simulink model "quadcoptermodel"  (R2017b)
settings: Solver=FixedStepAuto  StartTime=0.0  StopTime=11  FixedStep=1/250  RelTol=1e-3
values from neighbouring files (symbols this model uses):
  a1 = (Iyy-Izz)/Ixx    (= -1)    [param_init.m]
  a2 = Jr/Ixx    (= 0.00434930232558)    [param_init.m]
  a3 = (Izz-Ixx)/Iyy    (= 1)    [param_init.m]
  a4 = Jr/Iyy    (= 0.00434930232558)    [param_init.m]
  a5 = (Ixx-Iyy)/Izz    (= 0)    [param_init.m]
  b1 = l/Ixx    (= 26.1627906977)    [param_init.m]
  b2 = l/Iyy    (= 26.1627906977)    [param_init.m]
  b3 = l/Izz    (= 13.0813953488)    [param_init.m]
  g = 9.81    [param_init.m]
  kd_Phi = 0.1969    [param_init.m]
  kd_Psi = 0.1528    [param_init.m]
  kd_Theta = 0.2022    [param_init.m]
  kd_X = .7    (= 0.7)    [param_init.m]
  kd_Y = .7    (= 0.7)    [param_init.m]
  kd_Z = 10    [param_init.m]
  kf = 3.13e-5    (= 3.13e-05)    [param_init.m]
  ki_Phi = 2.2310    (= 2.231)    [param_init.m]
  ki_Psi = 1.8013    [param_init.m]
  ki_Theta = 2.1756    [param_init.m]
  ki_X = .1    (= 0.1)    [param_init.m]
  ki_Y = .1    (= 0.1)    [param_init.m]
  ki_Z = 0    [param_init.m]
  km = 9e-7    (= 9e-07)    [param_init.m]
  kp_Phi = 2.9996    [param_init.m]
  kp_Psi = 2.479    [param_init.m]
  kp_Theta = 3.0239    [param_init.m]
  kp_X = 2    [param_init.m]
  kp_Y = 2    [param_init.m]
  kp_Z = 30    [param_init.m]
  m = 0.4794    [param_init.m]
  omega_max = (90/100)*9000*(2*pi/(60))    (= 848.230016469)    [param_init.m]
libraries: simulink_extras x7, simulink x3, fuzblock x2, aerolibanim x1

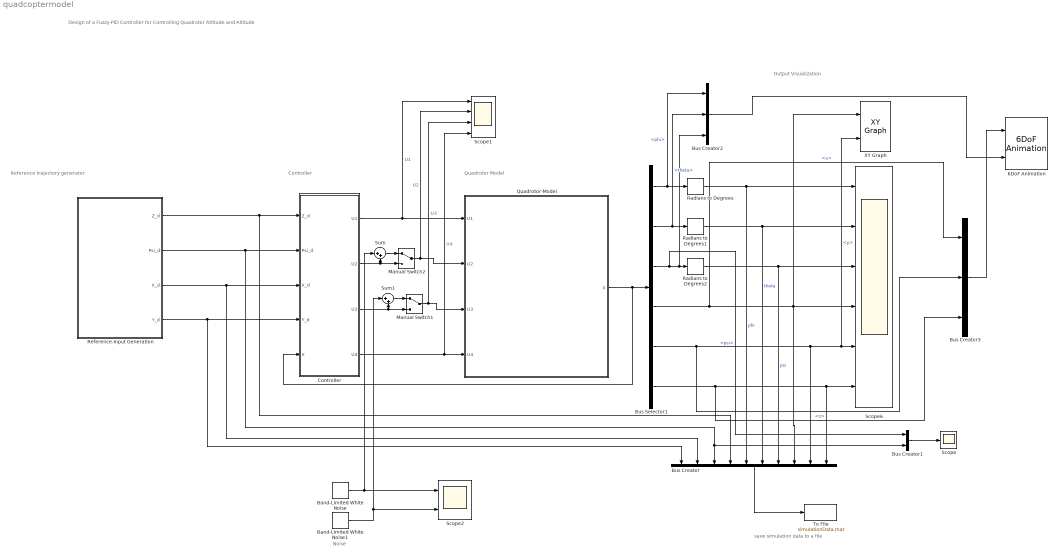
== system quadcoptermodel ==
  note: Noise
  note: Design of a Fuzzy-PID Controller for Controlling Quadrotor Attitude and Altitude
  note: save simulation data to a file
  note: Reference trajectory generator
  note: Output Visualization
  note: Controller
  note: Quadrotor Model
  6DoF Animation : aerolibanim/6DoF Animation  u1=[-2 2 -2 2 -1 3]  u2=0.1  u3=1  u4=[0 0 -10]  u5=Fixed position  u6=[10 2 -2]  u7=10  u8=on
  Band-Limited White Noise : simulink/Sources/Band-Limited White Noise  Cov=[0.1]  Ts=1  seed=[23341]
  Band-Limited White Noise1 : simulink/Sources/Band-Limited White Noise  Cov=[0.1]  Ts=1  seed=[23341]
  Bus Creator : BusCreator  Inputs=10
  Bus Creator1 : BusCreator  Inputs=2
  Bus Creator2 : BusCreator  Inputs=3
  Bus Creator3 : BusCreator  Inputs=3
  Bus Selector1 : BusSelector  OutputSignals=phi,theta,psi,x,y,z
  Controller : Subsystem
  Manual Switch1 : ManualSwitch
  Manual Switch2 : ManualSwitch
  Quadrotor-Model : Subsystem
  Radians to Degrees : simulink_extras/Transformations/Radians to Degrees
  Radians to Degrees1 : simulink_extras/Transformations/Radians to Degrees
  Radians to Degrees2 : simulink_extras/Transformations/Radians to Degrees
  Reference-Input Generation : Subsystem
  Scope : Scope
  Scope1 : Scope  NumInputPorts=4
  Scope2 : Scope  NumInputPorts=2
  Scope6 : Scope  NumInputPorts=6
  Sum : Sum  Inputs=|++
  Sum1 : Sum  Inputs=|++
  To File : ToFile  Filename=simulationData.mat  SaveFormat=Timeseries
  XY Graph : simulink/Sinks/XY Graph  xmin=-2  xmax=2  ymin=-2  ymax=2  st=-1
  wires:
  Bus Selector1/5 -> Bus Creator3/2, Bus Creator/9, XY Graph/2, Scope6/5  "<y>"
  Bus Selector1/6 -> Bus Creator3/3, Bus Creator/10, Scope6/6  "<z>"
  Bus Selector1/4 -> Bus Creator3/1, Bus Creator/8, XY Graph/1, Scope6/4  "<x>"
  Bus Selector1/1 -> Bus Creator2/1, Radians to Degrees/1  "<phi>"
  Radians to Degrees/1 -> Bus Creator/5, Scope6/1  "phi"
  Bus Selector1/2 -> Bus Creator2/2, Radians to Degrees1/1  "<theta>"
  Radians to Degrees1/1 -> Bus Creator/6, Scope6/2  "theta"
  Radians to Degrees2/1 -> Bus Creator/7, Scope6/3  "psi"
  Bus Selector1/3 -> Bus Creator1/1, Bus Creator2/3, Radians to Degrees2/1  "<psi>"
  Controller/4(U4) -> Scope1/4, Quadrotor-Model/4(U4)  "U4"
  Quadrotor-Model/1(X) -> Controller/5(X), Bus Selector1/1
  Reference-Input Generation/2(Psi_d) -> Bus Creator1/2, Bus Creator/3, Controller/2(Psi_d)
  Reference-Input Generation/3(X_d) -> Bus Creator/2, Controller/3(X_d)
  Bus Creator/1 -> To File/1
  Reference-Input Generation/1(Z_d) -> Bus Creator/4, Controller/1(Z_d)
  Reference-Input Generation/4(Y_d) -> Bus Creator/1, Controller/4(Y_d)
  Bus Creator1/1 -> Scope/1
  Controller/1(U1) -> Scope1/1, Quadrotor-Model/1(U1)  "U1"
  Manual Switch2/1 -> Scope1/2, Quadrotor-Model/2(U2)  "U2"
  Controller/2(U2) -> Sum/2, Manual Switch2/2
  Controller/3(U3) -> Sum1/2, Manual Switch1/2
  Manual Switch1/1 -> Scope1/3, Quadrotor-Model/3(U3)  "U3"
  Sum/1 -> Manual Switch2/1
  Band-Limited White Noise/1 -> Scope2/1, Sum/1
  Sum1/1 -> Manual Switch1/1
  Band-Limited White Noise1/1 -> Scope2/2, Sum1/1
  Bus Creator3/1 -> 6DoF Animation/1
  Bus Creator2/1 -> 6DoF Animation/2

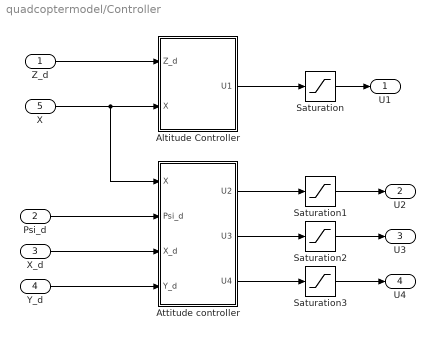
== system quadcoptermodel/Controller ==
  Z_d : Inport
  Psi_d : Inport  Port=2
  X_d : Inport  Port=3
  Y_d : Inport  Port=4
  X : Inport  Port=5
  Altitude Controller : Subsystem
  Attitude controller : Subsystem
  Saturation : Saturate  UpperLimit=91  LowerLimit=-91
  Saturation1 : Saturate  UpperLimit=23  LowerLimit=-23
  Saturation2 : Saturate  UpperLimit=23  LowerLimit=-23
  Saturation3 : Saturate  UpperLimit=1.3  LowerLimit=-1.3
  U1 : Outport
  U2 : Outport  Port=2
  U3 : Outport  Port=3
  U4 : Outport  Port=4
  wires:
  X/1 -> Attitude controller/1(X), Altitude Controller/2(X)
  Psi_d/1 -> Attitude controller/2(Psi_d)
  Z_d/1 -> Altitude Controller/1(Z_d)
  Y_d/1 -> Attitude controller/4(Y_d)
  X_d/1 -> Attitude controller/3(X_d)
  Altitude Controller/1(U1) -> Saturation/1
  Saturation/1 -> U1/1
  Saturation1/1 -> U2/1
  Attitude controller/1(U2) -> Saturation1/1
  Saturation2/1 -> U3/1
  Attitude controller/2(U3) -> Saturation2/1
  Saturation3/1 -> U4/1
  Attitude controller/3(U4) -> Saturation3/1

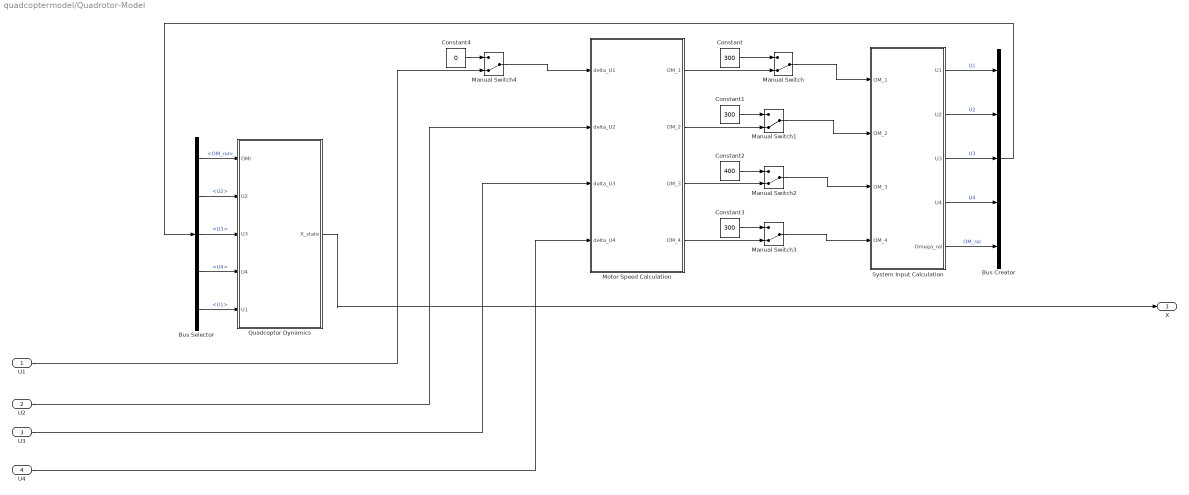
== system quadcoptermodel/Quadrotor-Model ==
  U1 : Inport
  U2 : Inport  Port=2
  U3 : Inport  Port=3
  U4 : Inport  Port=4
  Bus Creator : BusCreator  Inputs=5
  Bus Selector : BusSelector  OutputSignals=OM_rel,U2,U3,U4,U1
  Constant : Constant  Value=300
  Constant1 : Constant  Value=300
  Constant2 : Constant  Value=400
  Constant3 : Constant  Value=300
  Constant4 : Constant  Value=0
  Manual Switch{,1..4} (5 alike) : ManualSwitch  CurrentSetting=0
  Motor Speed Calculation : Subsystem
  Quadcoptor Dynamics : Subsystem
  System Input Calculation : Subsystem
  X : Outport
  wires:
  Constant/1 -> Manual Switch/1
  Bus Selector/2 -> Quadcoptor Dynamics/2(U2)  "<U2>"
  Bus Selector/4 -> Quadcoptor Dynamics/4(U4)  "<U4>"
  System Input Calculation/5(Omega_rel) -> Bus Creator/5  "OM_rel"
  System Input Calculation/3(U3) -> Bus Creator/3  "U3"
  Bus Selector/5 -> Quadcoptor Dynamics/5(U1)  "<U1>"
  Bus Creator/1 -> Bus Selector/1
  Bus Selector/3 -> Quadcoptor Dynamics/3(U3)  "<U3>"
  U3/1 -> Motor Speed Calculation/3(delta_U3)
  Manual Switch/1 -> System Input Calculation/1(OM_1)
  Manual Switch1/1 -> System Input Calculation/2(OM_2)
  U2/1 -> Motor Speed Calculation/2(delta_U2)
  Constant1/1 -> Manual Switch1/1
  Quadcoptor Dynamics/1(X_state) -> X/1
  Motor Speed Calculation/1(OM_1) -> Manual Switch/2
  Bus Selector/1 -> Quadcoptor Dynamics/1(OMr)  "<OM_rel>"
  System Input Calculation/1(U1) -> Bus Creator/1  "U1"
  U4/1 -> Motor Speed Calculation/4(delta_U4)
  System Input Calculation/4(U4) -> Bus Creator/4  "U4"
  System Input Calculation/2(U2) -> Bus Creator/2  "U2"
  Motor Speed Calculation/2(OM_2) -> Manual Switch1/2
  Motor Speed Calculation/4(OM_4) -> Manual Switch3/2
  Constant3/1 -> Manual Switch3/1
  Manual Switch2/1 -> System Input Calculation/3(OM_3)
  Constant2/1 -> Manual Switch2/1
  U1/1 -> Manual Switch4/2
  Manual Switch3/1 -> System Input Calculation/4(OM_4)
  Motor Speed Calculation/3(OM_3) -> Manual Switch2/2
  Constant4/1 -> Manual Switch4/1
  Manual Switch4/1 -> Motor Speed Calculation/1(delta_U1)

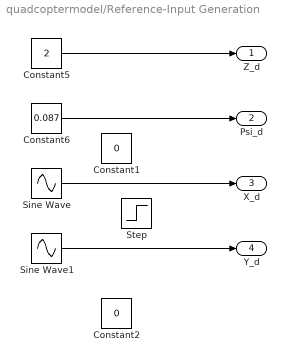
== system quadcoptermodel/Reference-Input Generation ==
  Constant1 : Constant  Value=0
  Constant2 : Constant  Value=0
  Constant5 : Constant  Value=2
  Constant6 : Constant  Value=0.087
  Sine Wave : Sin  SampleTime=0
  Sine Wave1 : Sin  Phase=pi/2  SampleTime=0
  Step : Step  After=.087  SampleTime=0
  Z_d : Outport
  Psi_d : Outport  Port=2
  X_d : Outport  Port=3
  Y_d : Outport  Port=4
  wires:
  Constant5/1 -> Z_d/1
  Constant6/1 -> Psi_d/1
  Sine Wave/1 -> X_d/1
  Sine Wave1/1 -> Y_d/1

== system quadcoptermodel/Controller/Altitude Controller ==
  Z_d : Inport
  X : Inport  Port=2
  AltitudeController : Subsystem
  Bus Selector : BusSelector  OutputSignals=z
  U1 : Outport
  wires:
  X/1 -> Bus Selector/1
  AltitudeController/1(U1) -> U1/1
  Bus Selector/1 -> AltitudeController/1(Z)  "<z>"
  Z_d/1 -> AltitudeController/2(Z_d)

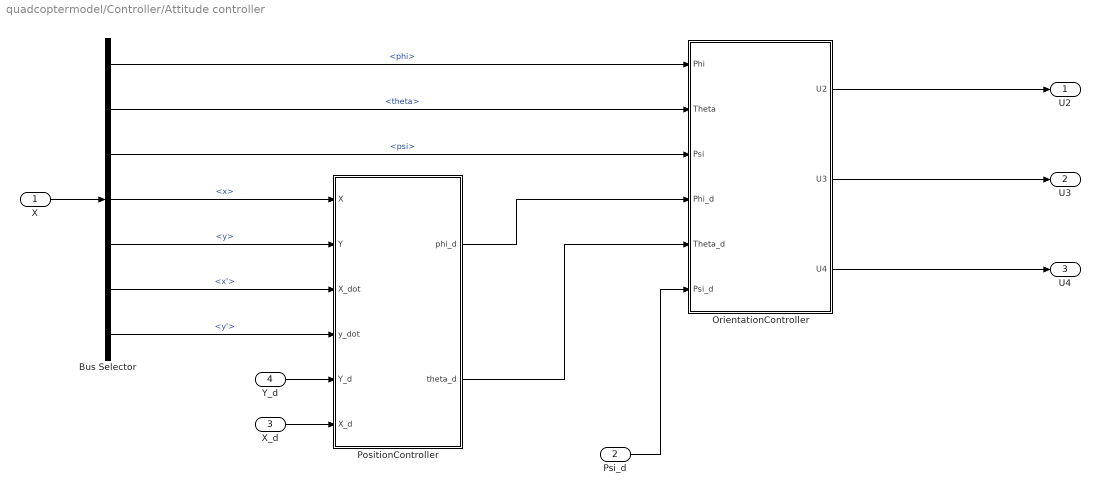
== system quadcoptermodel/Controller/Attitude controller ==
  X : Inport
  Psi_d : Inport  Port=2
  X_d : Inport  Port=3
  Y_d : Inport  Port=4
  Bus Selector : BusSelector  OutputSignals=phi,theta,psi,x,y,x',y'
  OrientationController : Subsystem
  PositionController : Subsystem
  U2 : Outport
  U3 : Outport  Port=2
  U4 : Outport  Port=3
  wires:
  Bus Selector/2 -> OrientationController/2(Theta)  "<theta>"
  Bus Selector/1 -> OrientationController/1(Phi)  "<phi>"
  Bus Selector/3 -> OrientationController/3(Psi)  "<psi>"
  OrientationController/1(U2) -> U2/1
  X/1 -> Bus Selector/1
  OrientationController/3(U4) -> U4/1
  OrientationController/2(U3) -> U3/1
  Bus Selector/4 -> PositionController/1(X)  "<x>"
  Bus Selector/5 -> PositionController/2(Y)  "<y>"
  Bus Selector/6 -> PositionController/3(X_dot)  "<x'>"
  Bus Selector/7 -> PositionController/4(y_dot)  "<y'>"
  Psi_d/1 -> OrientationController/6(Psi_d)
  X_d/1 -> PositionController/6(X_d)
  Y_d/1 -> PositionController/5(Y_d)
  PositionController/1(phi_d) -> OrientationController/4(Phi_d)
  PositionController/2(theta_d) -> OrientationController/5(Theta_d)

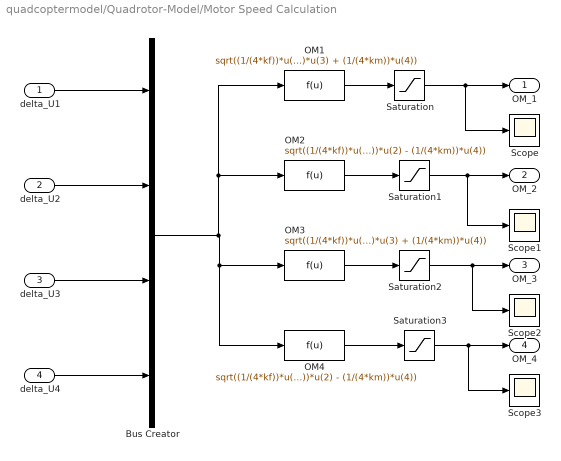
== system quadcoptermodel/Quadrotor-Model/Motor Speed Calculation ==
  delta_U1 : Inport
  delta_U2 : Inport  Port=2
  delta_U3 : Inport  Port=3
  delta_U4 : Inport  Port=4
  Bus Creator : BusCreator  Inputs=4
  OM1 : Fcn  Expr=sqrt((1/(4*kf))*u(1) + (1/(2*kf))*u(3) + (1/(4*km))*u(4))
  OM2 : Fcn  Expr=sqrt((1/(4*kf))*u(1) - (1/(2*kf))*u(2) - (1/(4*km))*u(4))
  OM3 : Fcn  Expr=sqrt((1/(4*kf))*u(1) - (1/(2*kf))*u(3) + (1/(4*km))*u(4))
  OM4 : Fcn  Expr=sqrt((1/(4*kf))*u(1) + (1/(2*kf))*u(2) - (1/(4*km))*u(4))
  Saturation{,1..3} (4 alike) : Saturate  UpperLimit=omega_max  LowerLimit=0
  Scope{,1..3} (4 alike) : Scope
  OM_1 : Outport
  OM_2 : Outport  Port=2
  OM_3 : Outport  Port=3
  OM_4 : Outport  Port=4
  wires:
  delta_U1/1 -> Bus Creator/1
  delta_U3/1 -> Bus Creator/3
  delta_U4/1 -> Bus Creator/4
  delta_U2/1 -> Bus Creator/2
  Bus Creator/1 -> OM2/1, OM1/1, OM3/1, OM4/1
  OM3/1 -> Saturation2/1
  OM2/1 -> Saturation1/1
  OM1/1 -> Saturation/1
  Saturation1/1 -> Scope1/1, OM_2/1
  Saturation2/1 -> Scope2/1, OM_3/1
  Saturation3/1 -> Scope3/1, OM_4/1
  OM4/1 -> Saturation3/1
  Saturation/1 -> Scope/1, OM_1/1

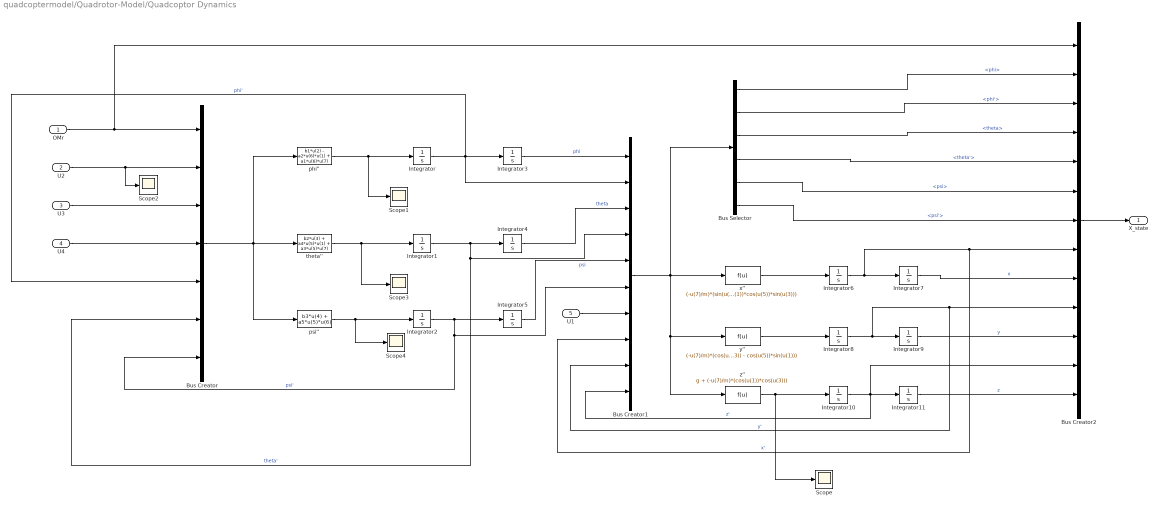
== system quadcoptermodel/Quadrotor-Model/Quadcoptor Dynamics ==
  OMr : Inport
  U2 : Inport  Port=2
  U3 : Inport  Port=3
  U4 : Inport  Port=4
  U1 : Inport  Port=5
  Bus Creator : BusCreator  Inputs=7
  Bus Creator1 : BusCreator  Inputs=10
  Bus Creator2 : BusCreator  Inputs=13
  Bus Selector : BusSelector  OutputSignals=phi,phi',theta,theta',psi,psi'
  Integrator{,1..11} (12 alike) : Integrator
  Scope{,1..4} (5 alike) : Scope
  phi'' : Fcn  Expr=b1*u(2) - a2*u(6)*u(1) + a1*u(6)*u(7)
  psi'' : Fcn  Expr=b3*u(4) + a5*u(5)*u(6)
  theta'' : Fcn  Expr=b2*u(3) + a4*u(5)*u(1) + a3*u(5)*u(7)
  x'' : Fcn  Expr=(-u(7)/m)*(sin(u(1))*sin(u(5)) + cos(u(1))*cos(u(5))*sin(u(3)))
  y'' : Fcn  Expr=(-u(7)/m)*(cos(u(1))*sin(u(5))*sin(u(3)) - cos(u(5))*sin(u(1)))
  z'' : Fcn  Expr=g + (-u(7)/m)*(cos(u(1))*cos(u(3)))
  X_state : Outport
  wires:
  U1/1 -> Bus Creator1/7
  OMr/1 -> Bus Creator2/1, Bus Creator/1
  Integrator7/1 -> Bus Creator2/9  "x"
  Bus Creator/1 -> psi''/1, phi''/1, theta''/1
  Bus Creator2/1 -> X_state/1
  psi''/1 -> Scope4/1, Integrator2/1
  Integrator10/1 -> Bus Creator1/10, Bus Creator2/12, Integrator11/1  "z'"
  Integrator1/1 -> Bus Creator/6, Bus Creator1/4, Integrator4/1  "theta'"
  Integrator4/1 -> Bus Creator1/3  "theta"
  Integrator11/1 -> Bus Creator2/13  "z"
  Integrator/1 -> Bus Creator1/2, Bus Creator/5, Integrator3/1  "phi'"
  Integrator5/1 -> Bus Creator1/5  "psi"
  Bus Selector/6 -> Bus Creator2/7  "<psi'>"
  Integrator6/1 -> Bus Creator1/8, Bus Creator2/8, Integrator7/1  "x'"
  U2/1 -> Scope2/1, Bus Creator/2
  Integrator3/1 -> Bus Creator1/1  "phi"
  U4/1 -> Bus Creator/4
  Integrator9/1 -> Bus Creator2/11  "y"
  theta''/1 -> Scope3/1, Integrator1/1
  Bus Selector/1 -> Bus Creator2/2  "<phi>"
  y''/1 -> Integrator8/1
  z''/1 -> Scope/1, Integrator10/1
  Integrator2/1 -> Bus Creator1/6, Bus Creator/7, Integrator5/1  "psi'"
  U3/1 -> Bus Creator/3
  Bus Selector/2 -> Bus Creator2/3  "<phi'>"
  Bus Selector/4 -> Bus Creator2/5  "<theta'>"
  Bus Selector/5 -> Bus Creator2/6  "<psi>"
  x''/1 -> Integrator6/1
  phi''/1 -> Scope1/1, Integrator/1
  Integrator8/1 -> Bus Creator1/9, Bus Creator2/10, Integrator9/1  "y'"
  Bus Creator1/1 -> y''/1, z''/1, Bus Selector/1, x''/1
  Bus Selector/3 -> Bus Creator2/4  "<theta>"

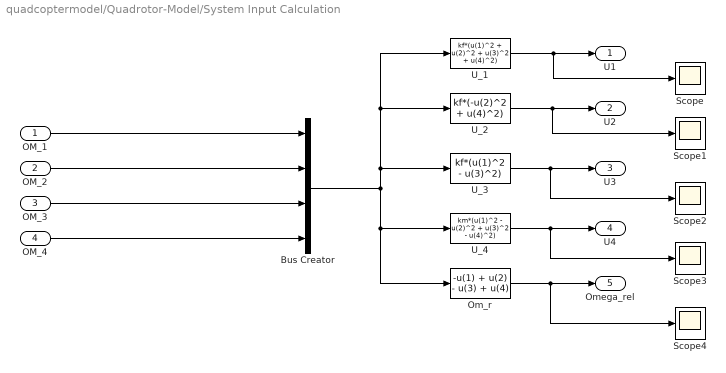
== system quadcoptermodel/Quadrotor-Model/System Input Calculation ==
  OM_1 : Inport
  OM_2 : Inport  Port=2
  OM_3 : Inport  Port=3
  OM_4 : Inport  Port=4
  Bus Creator : BusCreator  Inputs=4
  Om_r : Fcn  Expr=-u(1) + u(2) - u(3) + u(4)
  Scope{,1..4} (5 alike) : Scope
  U_1 : Fcn  Expr=kf*(u(1)^2 + u(2)^2 + u(3)^2 + u(4)^2)
  U_2 : Fcn  Expr=kf*(-u(2)^2 + u(4)^2)
  U_3 : Fcn  Expr="kf*(u(1)^2  - u(3)^2)"
  U_4 : Fcn  Expr=km*(u(1)^2 - u(2)^2 + u(3)^2 - u(4)^2)
  U1 : Outport
  U2 : Outport  Port=2
  U3 : Outport  Port=3
  U4 : Outport  Port=4
  Omega_rel : Outport  Port=5
  wires:
  Om_r/1 -> Scope4/1, Omega_rel/1
  U_4/1 -> Scope3/1, U4/1
  U_1/1 -> Scope/1, U1/1
  U_2/1 -> Scope1/1, U2/1
  U_3/1 -> Scope2/1, U3/1
  Bus Creator/1 -> U_2/1, U_1/1, U_3/1, U_4/1, Om_r/1
  OM_1/1 -> Bus Creator/1
  OM_2/1 -> Bus Creator/2
  OM_3/1 -> Bus Creator/3
  OM_4/1 -> Bus Creator/4

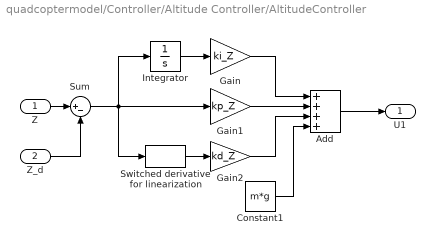
== system quadcoptermodel/Controller/Altitude Controller/AltitudeController ==
  Z : Inport
  Z_d : Inport  Port=2
  Add : Sum  Inputs=++++
  Constant1 : Constant  Value=m*g
  Gain : Gain  Gain=ki_Z
  Gain1 : Gain  Gain=kp_Z
  Gain2 : Gain  Gain=kd_Z
  Integrator : Integrator
  Sum : Sum  Inputs=|+-
  Switched derivative for linearization : simulink_extras/Linearization/Switched derivative for linearization  switchVal=1  derivConst=100
  U1 : Outport
  wires:
  Integrator/1 -> Gain/1
  Gain2/1 -> Add/3
  Gain/1 -> Add/1
  Gain1/1 -> Add/2
  Sum/1 -> Switched derivative for linearization/1, Gain1/1, Integrator/1
  Z/1 -> Sum/1
  Add/1 -> U1/1
  Switched derivative for linearization/1 -> Gain2/1
  Z_d/1 -> Sum/2
  Constant1/1 -> Add/4

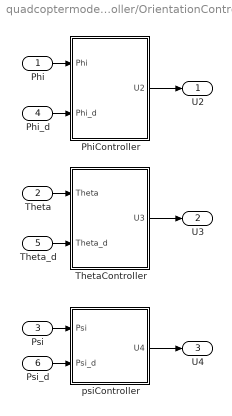
== system quadcoptermodel/Controller/Attitude controller/OrientationController ==
  Phi : Inport
  Theta : Inport  Port=2
  Psi : Inport  Port=3
  Phi_d : Inport  Port=4
  Theta_d : Inport  Port=5
  Psi_d : Inport  Port=6
  PhiController : Subsystem
  ThetaController : Subsystem
  psiController : Subsystem
  U2 : Outport
  U3 : Outport  Port=2
  U4 : Outport  Port=3
  wires:
  Phi/1 -> PhiController/1(Phi)
  PhiController/1(U2) -> U2/1
  ThetaController/1(U3) -> U3/1
  psiController/1(U4) -> U4/1
  Psi/1 -> psiController/1(Psi)
  Theta/1 -> ThetaController/1(Theta)
  Theta_d/1 -> ThetaController/2(Theta_d)
  Phi_d/1 -> PhiController/2(Phi_d)
  Psi_d/1 -> psiController/2(Psi_d)

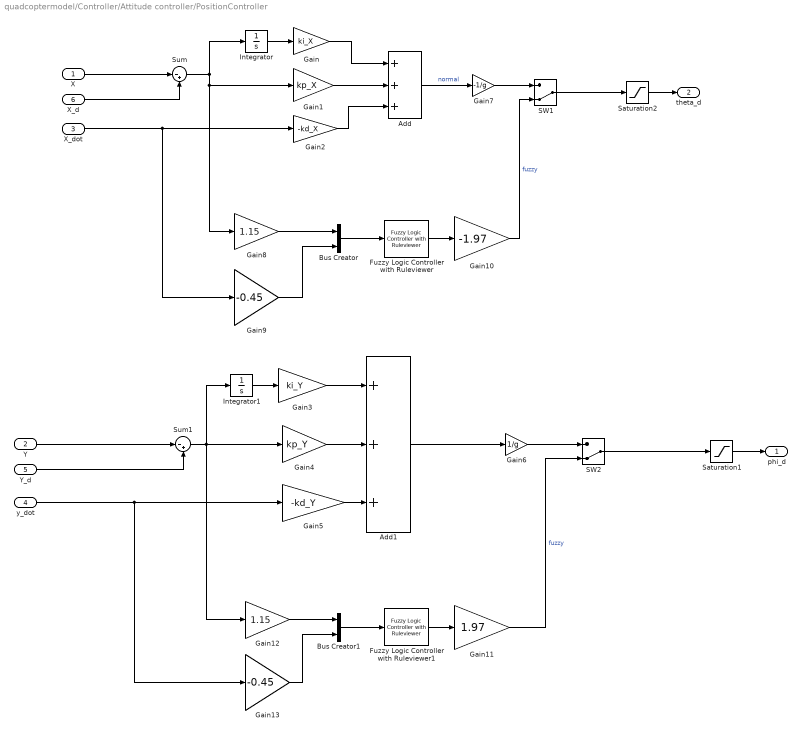
== system quadcoptermodel/Controller/Attitude controller/PositionController ==
  X : Inport
  Y : Inport  Port=2
  X_dot : Inport  Port=3
  y_dot : Inport  Port=4
  Y_d : Inport  Port=5
  X_d : Inport  Port=6
  Add : Sum  Inputs=+++
  Add1 : Sum  Inputs=+++
  Bus Creator : BusCreator  Inputs=2
  Bus Creator1 : BusCreator  Inputs=2
  Fuzzy Logic Controller with Ruleviewer : fuzblock/Fuzzy Logic  Controller  with Ruleviewer  fismatrix=quadrotorXY_fis  Ts=1
  Fuzzy Logic Controller with Ruleviewer1 : fuzblock/Fuzzy Logic  Controller  with Ruleviewer  fismatrix=quadrotorXY_fis  Ts=1
  Gain : Gain  Gain=ki_X
  Gain1 : Gain  Gain=kp_X
  Gain10 : Gain  Gain=-1.97
  Gain11 : Gain  Gain=1.97
  Gain12 : Gain  Gain=1.15
  Gain13 : Gain  Gain=-0.45
  Gain2 : Gain  Gain=-kd_X
  Gain3 : Gain  Gain=ki_Y
  Gain4 : Gain  Gain=kp_Y
  Gain5 : Gain  Gain=-kd_Y
  Gain6 : Gain  Gain=1/g
  Gain7 : Gain  Gain=-1/g
  Gain8 : Gain  Gain=1.15
  Gain9 : Gain  Gain=-0.45
  Integrator : Integrator
  Integrator1 : Integrator
  SW1 : ManualSwitch  CurrentSetting=0
  SW2 : ManualSwitch  CurrentSetting=0
  Saturation1 : Saturate  UpperLimit=0.3  LowerLimit=-0.3
  Saturation2 : Saturate  UpperLimit=0.3  LowerLimit=-0.3
  Sum : Sum  Inputs=|-+
  Sum1 : Sum  Inputs=|-+
  phi_d : Outport
  theta_d : Outport  Port=2
  wires:
  Y_d/1 -> Sum1/2
  X_d/1 -> Sum/2
  Integrator1/1 -> Gain3/1
  Gain4/1 -> Add1/2
  Gain3/1 -> Add1/1
  Gain5/1 -> Add1/3
  X/1 -> Sum/1
  Y/1 -> Sum1/1
  Integrator/1 -> Gain/1
  Sum/1 -> Gain8/1, Gain1/1, Integrator/1
  Gain1/1 -> Add/2
  Gain/1 -> Add/1
  Gain2/1 -> Add/3
  X_dot/1 -> Gain9/1, Gain2/1
  y_dot/1 -> Gain13/1, Gain5/1
  Saturation1/1 -> phi_d/1
  Saturation2/1 -> theta_d/1
  Add/1 -> Gain7/1  "normal"
  Bus Creator/1 -> Fuzzy Logic Controller with Ruleviewer/1
  Gain9/1 -> Bus Creator/2
  Gain8/1 -> Bus Creator/1
  Fuzzy Logic Controller with Ruleviewer/1 -> Gain10/1
  Gain10/1 -> SW1/2  "fuzzy"
  Fuzzy Logic Controller with Ruleviewer1/1 -> Gain11/1
  Gain13/1 -> Bus Creator1/2
  Sum1/1 -> Gain12/1, Gain4/1, Integrator1/1
  Gain12/1 -> Bus Creator1/1
  Bus Creator1/1 -> Fuzzy Logic Controller with Ruleviewer1/1
  Gain11/1 -> SW2/2  "fuzzy"
  SW1/1 -> Saturation2/1
  Gain7/1 -> SW1/1
  Gain6/1 -> SW2/1
  SW2/1 -> Saturation1/1
  Add1/1 -> Gain6/1

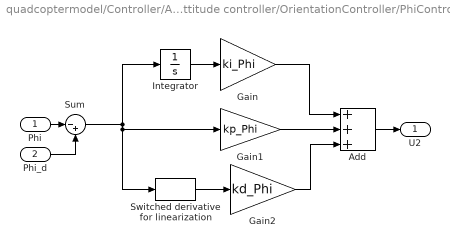
== system quadcoptermodel/Controller/Attitude controller/OrientationController/PhiController ==
  Phi : Inport
  Phi_d : Inport  Port=2
  Add : Sum  Inputs=+++
  Gain : Gain  Gain=ki_Phi
  Gain1 : Gain  Gain=kp_Phi
  Gain2 : Gain  Gain=kd_Phi
  Integrator : Integrator
  Sum : Sum  Inputs=|-+
  Switched derivative for linearization : simulink_extras/Linearization/Switched derivative for linearization  switchVal=1  derivConst=100
  U2 : Outport
  wires:
  Integrator/1 -> Gain/1
  Gain2/1 -> Add/3
  Gain/1 -> Add/1
  Gain1/1 -> Add/2
  Switched derivative for linearization/1 -> Gain2/1
  Phi/1 -> Sum/1
  Add/1 -> U2/1
  Sum/1 -> Gain1/1, Switched derivative for linearization/1, Integrator/1
  Phi_d/1 -> Sum/2

== system quadcoptermodel/Controller/Attitude controller/OrientationController/ThetaController ==
  Theta : Inport
  Theta_d : Inport  Port=2
  Add : Sum  Inputs=+++
  Gain : Gain  Gain=ki_Theta
  Gain1 : Gain  Gain=kp_Theta
  Gain2 : Gain  Gain=kd_Theta
  Integrator : Integrator
  Sum : Sum  Inputs=|-+
  Switched derivative for linearization : simulink_extras/Linearization/Switched derivative for linearization  switchVal=1  derivConst=100
  U3 : Outport
  wires:
  Integrator/1 -> Gain/1
  Gain2/1 -> Add/3
  Gain/1 -> Add/1
  Gain1/1 -> Add/2
  Switched derivative for linearization/1 -> Gain2/1
  Theta/1 -> Sum/1
  Add/1 -> U3/1
  Sum/1 -> Switched derivative for linearization/1, Gain1/1, Integrator/1
  Theta_d/1 -> Sum/2

== system quadcoptermodel/Controller/Attitude controller/OrientationController/psiController ==
  Psi : Inport
  Psi_d : Inport  Port=2
  Add : Sum  Inputs=+++
  Gain : Gain  Gain=ki_Psi
  Gain1 : Gain  Gain=kp_Psi
  Gain2 : Gain  Gain=kd_Psi
  Integrator : Integrator
  Sum : Sum  Inputs=|-+
  Switched derivative for linearization : simulink_extras/Linearization/Switched derivative for linearization  switchVal=1  derivConst=100
  U4 : Outport
  wires:
  Integrator/1 -> Gain/1
  Gain2/1 -> Add/3
  Gain/1 -> Add/1
  Gain1/1 -> Add/2
  Switched derivative for linearization/1 -> Gain2/1
  Psi/1 -> Sum/1
  Add/1 -> U4/1
  Psi_d/1 -> Sum/2
  Sum/1 -> Integrator/1, Switched derivative for linearization/1, Gain1/1
